simulink library "INT_StSys_StrtCtl"  (R2016b)
settings: Solver=VariableStepAuto  StartTime=0.0  StopTime=10.0  RelTol=1e-3
settings Model: Creator=xuxingpei  LastModifiedBy=xuxingpei

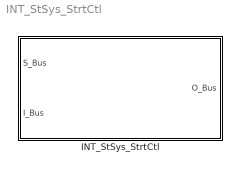
== system INT_StSys_StrtCtl ==
  INT_StSys_StrtCtl : Subsystem

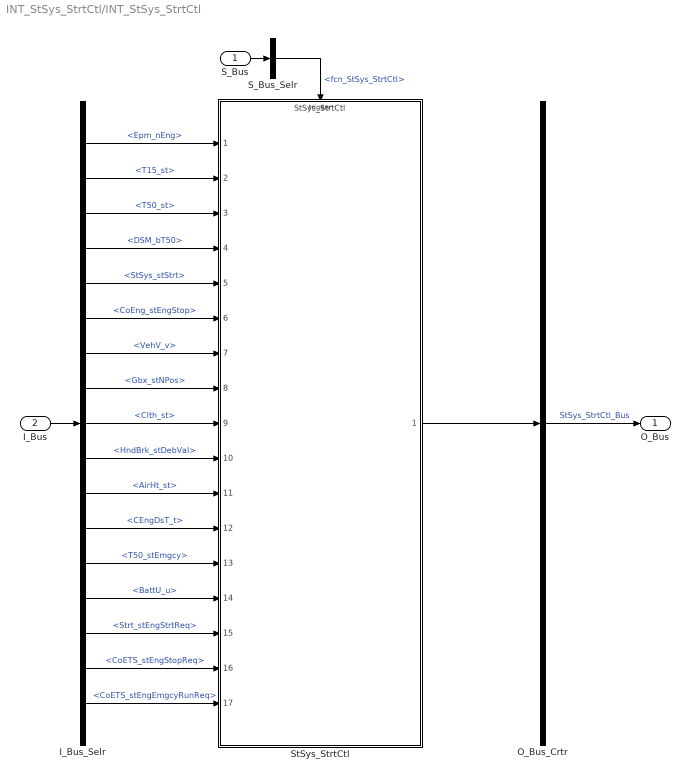
== system INT_StSys_StrtCtl/INT_StSys_StrtCtl ==
  S_Bus : Inport
  I_Bus : Inport  Port=2
  I_Bus_Selr : BusSelector  OutputSignals=Epm_nEng,T15_st,T50_st,DSM_bT50,StSys_stStrt,CoEng_stEngStop,VehV_v,Gbx_stNPos,Clth_st,HndBrk_stDebVal,AirHt_st,CEngDsT_t,T50_stEmgcy,BattU_u,Strt_stEngStrtReq,CoETS_stEngStopReq,CoETS_stEngEmgcyRunReq
  O_Bus_Crtr : BusCreator  Inputs=1
  S_Bus_Selr : BusSelector  OutputSignals=fcn_StSys_StrtCtl
  StSys_StrtCtl : ModelReference  ModelNameDialog=StSys_StrtCtl  SimulationMode=Normal  ModelReferenceVersion=1.588  TriggerPortName=function  TriggerPortTriggerType=function-call  TriggerPortStatesWhenEnabling=held
  O_Bus : Outport
  wires:
  S_Bus_Selr/1 -> StSys_StrtCtl/Trigger  "<fcn_StSys_StrtCtl>"
  S_Bus/1 -> S_Bus_Selr/1
  I_Bus/1 -> I_Bus_Selr/1
  I_Bus_Selr/1 -> StSys_StrtCtl/1  "<Epm_nEng>"
  I_Bus_Selr/2 -> StSys_StrtCtl/2  "<T15_st>"
  I_Bus_Selr/3 -> StSys_StrtCtl/3  "<T50_st>"
  I_Bus_Selr/4 -> StSys_StrtCtl/4  "<DSM_bT50>"
  I_Bus_Selr/5 -> StSys_StrtCtl/5  "<StSys_stStrt>"
  I_Bus_Selr/6 -> StSys_StrtCtl/6  "<CoEng_stEngStop>"
  I_Bus_Selr/7 -> StSys_StrtCtl/7  "<VehV_v>"
  I_Bus_Selr/8 -> StSys_StrtCtl/8  "<Gbx_stNPos>"
  I_Bus_Selr/9 -> StSys_StrtCtl/9  "<Clth_st>"
  I_Bus_Selr/10 -> StSys_StrtCtl/10  "<HndBrk_stDebVal>"
  I_Bus_Selr/11 -> StSys_StrtCtl/11  "<AirHt_st>"
  I_Bus_Selr/12 -> StSys_StrtCtl/12  "<CEngDsT_t>"
  I_Bus_Selr/13 -> StSys_StrtCtl/13  "<T50_stEmgcy>"
  I_Bus_Selr/14 -> StSys_StrtCtl/14  "<BattU_u>"
  I_Bus_Selr/15 -> StSys_StrtCtl/15  "<Strt_stEngStrtReq>"
  I_Bus_Selr/16 -> StSys_StrtCtl/16  "<CoETS_stEngStopReq>"
  I_Bus_Selr/17 -> StSys_StrtCtl/17  "<CoETS_stEngEmgcyRunReq>"
  O_Bus_Crtr/1 -> O_Bus/1  "StSys_StrtCtl_Bus"
  StSys_StrtCtl/1 -> O_Bus_Crtr/1
